simulink model "TwoDSimSimpleAero1stGen"  (R2021b)
settings: Solver=VariableStepAuto  StartTime=0.0  StopTime=5  RelTol=1e-3
undefined symbols (not defined in the file): Dterm, Iterm, Pterm
libraries: simulink_extras x4, simulink x1, slpidlib x1
settings Model: Creator=Andres  LastModifiedBy=Andres
settings SolverCC: ZeroCrossAlgorithm=Adaptive
settings DebuggingCC: AlgebraicLoopMsg=none  IgnoredZcDiagnostic=none

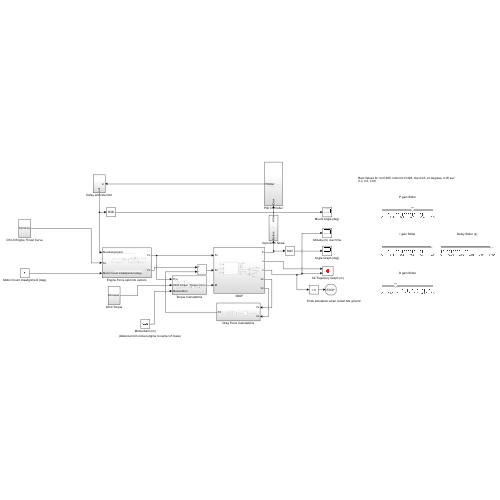
[thumbnail: Simulink's stored preview of the top-level diagram]
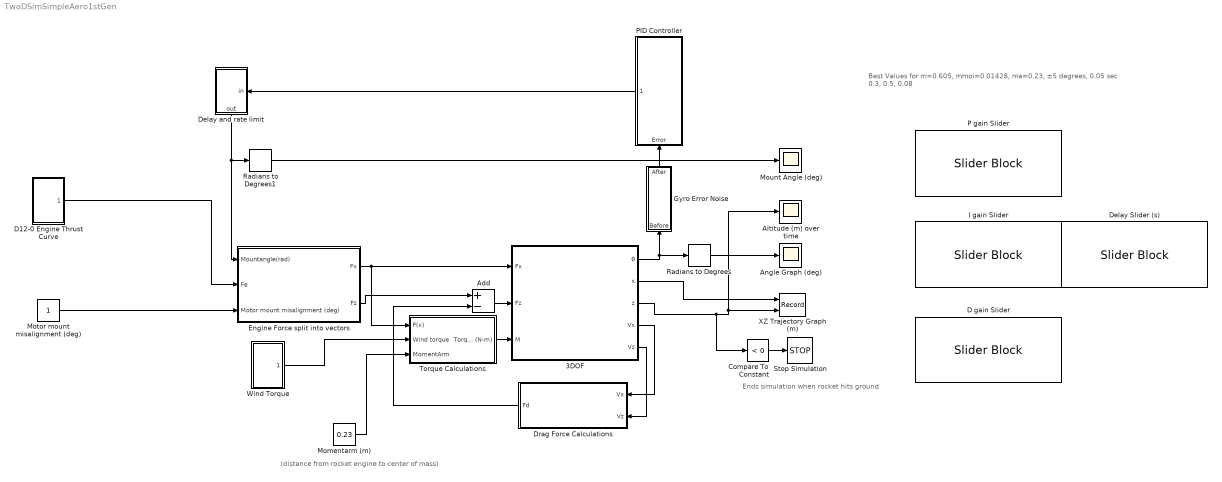
== system TwoDSimSimpleAero1stGen ==
  note: Best Values for m=0.605, mmoi=0.01428, ma=0.23, ±5 degrees, 0.05 sec
      | 0.3, 0.5, 0.08
  note: Ends simulation when rocket hits ground
  note: (distance from rocket engine to center of mass)
  3DOF : Subsystem
  Add : Sum  Inputs=+-
  Altitude (m) over time : Scope
  Angle Graph (deg) : Scope
  Compare To Constant : simulink/Logic and Bit Operations/Compare To Constant  relop=<  const=0  OutDataTypeStr=boolean
  D gain Slider : SliderBlock  LabelPosition=Hide  ScaleMax=0.3
  D12-0 Engine Thrust Curve : Subsystem
  Delay Slider (s) : SliderBlock  LabelPosition=Hide  ScaleMax=0.05  TickInterval=0.01
  Delay and rate limit : Subsystem
      settings: PortSchema="{\"entries\":[{\"content\":{\"sides\":[{\"content\":{\"connectorIds\":[\"In1\"]},\"type\":\"ConnectorPlacement.EquallySpacedRectSide\",\"uuid\":\"7f945310-91d5-4a5b-a152-cb378cea97e0\"},{\"content\":{\"connectorIds\":[],\"side\":\"RIGHT\"},\"type\":\"ConnectorPlacement.EquallySpacedRectSide\",\"uuid\":\"570eb395-808b-402d-8169-834796957515\"},{\"content\":{\"connectorIds\":[],\"side\":\"TOP\"},\"type\":\"ConnectorPlacement.EquallySpacedRectSide\",\"uuid\":\"f414d9f5-06db-41f9-9870-e73b040f5e14\"},{\"content\":{\"connectorIds\":[\"Out1\"],\"side\":\"BOTTOM\"},\"type\":\"ConnectorPlacement.EquallySpacedRectSide\",\"uuid\":\"dd3ad95d-53d5-4309-a4ef-7403eee50954\"}]},\"type\":\"ConnectorPlacement.EquallySpacedConnector\",\"uuid\":\"16f64462-feef-497e-ac9f-2db815891e61\"}],\"packageUris\":[\"http://schema.mathworks.com/mf0/Connector/R2020b\"],\"version\":\"1.0\"}"
  Drag Force Calculations : Subsystem
  Engine Force split into vectors : Subsystem
  Gyro Error Noise : Subsystem
      settings: PortSchema="{\"entries\":[{\"content\":{\"sides\":[{\"content\":{\"connectorIds\":[]},\"type\":\"ConnectorPlacement.EquallySpacedRectSide\",\"uuid\":\"db613b74-a95a-4e78-b0b5-852c38ce090d\"},{\"content\":{\"connectorIds\":[],\"side\":\"RIGHT\"},\"type\":\"ConnectorPlacement.EquallySpacedRectSide\",\"uuid\":\"8ff7bb38-cc09-4562-ae4b-2277c61965ca\"},{\"content\":{\"connectorIds\":[\"Out1\"],\"side\":\"TOP\"},\"type\":\"ConnectorPlacement.EquallySpacedRectSide\",\"uuid\":\"fa7b536e-f18b-43ee-b35a-7562f98f0dcc\"},{\"content\":{\"connectorIds\":[\"In1\"],\"side\":\"BOTTOM\"},\"type\":\"ConnectorPlacement.EquallySpacedRectSide\",\"uuid\":\"dd72ef68-23e3-4e8c-8031-36f0d8372741\"}]},\"type\":\"ConnectorPlacement.EquallySpacedConnector\",\"uuid\":\"56970b38-3c02-4837-94fb-dc8b3090c774\"}],\"packageUris\":[\"http://schema.mathworks.com/mf0/Connector/R2020b\"],\"version\":\"1.0\"}"
  I gain Slider : SliderBlock  LabelPosition=Hide  ScaleMax=0.5
  Momentarm (m) : Constant  Value=0.23
  Motor mount misalignment (deg) : Constant
  Mount Angle (deg) : Scope
  P gain Slider : SliderBlock  LabelPosition=Hide  ScaleMax=0.5
  PID Controller : Subsystem
      settings: PortSchema="{\"entries\":[{\"content\":{\"sides\":[{\"content\":{\"connectorIds\":[\"Out1\"]},\"type\":\"ConnectorPlacement.EquallySpacedRectSide\",\"uuid\":\"3056940d-b626-4ad3-aea6-cbabeac63329\"},{\"content\":{\"connectorIds\":[],\"side\":\"RIGHT\"},\"type\":\"ConnectorPlacement.EquallySpacedRectSide\",\"uuid\":\"0510cd9b-8fa4-4f8a-80ec-38231d972233\"},{\"content\":{\"connectorIds\":[],\"side\":\"TOP\"},\"type\":\"ConnectorPlacement.EquallySpacedRectSide\",\"uuid\":\"9c9a70ab-b090-41d6-ac7a-a7598bc3d7a5\"},{\"content\":{\"connectorIds\":[\"In1\"],\"side\":\"BOTTOM\"},\"type\":\"ConnectorPlacement.EquallySpacedRectSide\",\"uuid\":\"76047b82-5909-4180-a207-d443029300af\"}]},\"type\":\"ConnectorPlacement.EquallySpacedConnector\",\"uuid\":\"ba61792f-c506-461f-9738-365393edbd5c\"}],\"packageUris\":[\"http://schema.mathworks.com/mf0/Connector/R2020b\"],\"version\":\"1.0\"}"
  Radians to Degrees : simulink_extras/Transformations/Radians to Degrees
  Radians to Degrees1 : simulink_extras/Transformations/Radians to Degrees
  Stop Simulation : Stop
  Torque Calculations : Subsystem
  Wind Torque : Subsystem
  XZ Trajectory Graph (m) : Record  FileSettingsInternal="{\"entries\":[{\"content\":{\"excelSettings\":{\"content\":{},\"type\":\"Streamout.ExcelSettings\"}},\"type\":\"Streamout.FileSettingStorage\",\"uuid\":\"b17d18d2-045f-4c2f-bb1f-32f760d49c3f\"}],\"packageUris\":[\"http://schema.mathworks.com/mf0/streamout_blocks/R2020a\"],\"version\":\"1.0\"}"  Layout=[1 1]  SignalsInternal="{\"entries\":[{\"content\":{\"signals\":[{\"content\":{\"blockPath\":[\"TwoDSimSimpleAero1stGen/XZ Trajectory Graph (m)\"],\"channel\":[],\"dimensions\":[1],\"domain\":\"TwoDSimSimpleAero1stGen/XZ Trajectory Graph (m)\",\"lineColor\":\"#fe330a\",\"plots\":[1],\"port\":1,\"sid\":[\"\"],\"signalID\":81,\"signalName\":\"3DOF:2\"},\"type\":\"RecordBlkView.Signal\",\"uuid\":\"15905c86-6a6c-439f-aa8f-17a391bc4a57\"},{\"content\":{\"blockPath\":[\"TwoDSimSimpleAero1stGen/XZ Trajectory Graph (m)\"],\"channel\":[],\"dimensions\":[1],\"domain\":\"TwoDSimSimpleAero1stGen/XZ Trajectory Graph (m)\",\"lineColor\":\"#22b573\",\"plots\":[1],\"port\":2,\"sid\":[\"\"],\"signalID\":85,\"signalName\":\"3DOF:3\"},\"type\":\"RecordBlkView.Signal\",\"uuid\":\"f1bda5b5-dd59-48e2-bdf2-818b15901255\"}]},\"type\":\"RecordBlkView.InputSignals\",\"uuid\":\"d9778f91-fdcf-43d5-b0d8-99f691514bf1\"}],\"packageUris\":[\"http://schema.mathworks.com/mf0/streamout_blocks/R2020a\"],\"version\":\"1.0\"}"  VisualizationBindings="{\"xyplotplugin\":{\"info\":[{\"series\":[{\"bindingParametersList\":[{\"parameter\":\"X-Axis\",\"signalID\":81,\"signalName\":\"3DOF:2\"},{\"parameter\":\"Y-Axis\",\"signalID\":85,\"signalName\":\"3DOF:3\"}],\"seriesID\":63584}],\"subplotID\":1}]}}"  CompatibilityTag=XY
  wires:
  3DOF/3(z) -> Altitude (m) over time/1, XZ Trajectory Graph (m)/2, Compare To Constant/1
  Compare To Constant/1 -> Stop Simulation/1
  3DOF/2(x) -> XZ Trajectory Graph (m)/1
  Motor mount misalignment (deg)/1 -> Engine Force split into vectors/3(Motor mount misalignment (deg))
  D12-0 Engine Thrust Curve/1(F(D12-0)) -> Engine Force split into vectors/2(Fe)
  Gyro Error Noise/1(After) -> PID Controller/1(Error)
  Delay and rate limit/1(out) -> Engine Force split into vectors/1(Mountangle(rad)), Radians to Degrees1/1
  Momentarm (m)/1 -> Torque Calculations/3(MomentArm)
  Radians to Degrees1/1 -> Mount Angle (deg)/1
  Engine Force split into vectors/2(Fz) -> Add/1
  Engine Force split into vectors/1(Fx) -> 3DOF/1(Fx), Torque Calculations/1(F(x))
  Drag Force Calculations/1(Fd) -> Add/2
  3DOF/1(" θ") -> Radians to Degrees/1, Gyro Error Noise/1(Before)
  Add/1 -> 3DOF/2(Fz)
  Torque Calculations/1(Torque (N-m)) -> 3DOF/3(M)
  3DOF/4(Vx) -> Drag Force Calculations/1(Vx)
  3DOF/5(Vz) -> Drag Force Calculations/2(Vz)
  Radians to Degrees/1 -> Angle Graph (deg)/1
  PID Controller/1(PIDOut) -> Delay and rate limit/1(in)
  Wind Torque/1(Wind torque) -> Torque Calculations/2(Wind torque)

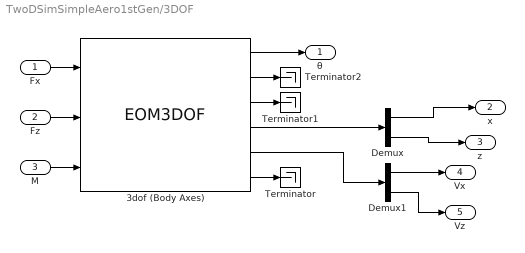
== system TwoDSimSimpleAero1stGen/3DOF ==
  Fx : Inport
  Fz : Inport  Port=2
  M : Inport  Port=3
  3dof (Body Axes) : EOM3DOF  v_ini=0.00000000000000000001  pos_ini=[0 0.1]  mass=0.605  Iyy=0.01428  g=-9.81
  Demux : Demux  Outputs=2
  Demux1 : Demux  Outputs=2
  Terminator : Terminator
  Terminator1 : Terminator
  Terminator2 : Terminator
  " θ" : Outport
  x : Outport  Port=2
  z : Outport  Port=3
  Vx : Outport  Port=4
  Vz : Outport  Port=5
  wires:
  Fz/1 -> 3dof (Body Axes)/2
  3dof (Body Axes)/2 -> Terminator2/1
  3dof (Body Axes)/6 -> Terminator/1
  Fx/1 -> 3dof (Body Axes)/1
  3dof (Body Axes)/3 -> Terminator1/1
  M/1 -> 3dof (Body Axes)/3
  3dof (Body Axes)/1 -> " θ"/1
  3dof (Body Axes)/4 -> Demux/1
  Demux/1 -> x/1
  Demux/2 -> z/1
  3dof (Body Axes)/5 -> Demux1/1
  Demux1/1 -> Vx/1
  Demux1/2 -> Vz/1

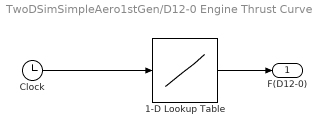
== system TwoDSimSimpleAero1stGen/D12-0 Engine Thrust Curve ==
  1-D Lookup Table : Lookup_n-D  NumberOfTableDimensions=1  BreakpointsForDimension1=[0 0.049 0.116 0.184 0.237 0.282 0.297 0.311 0.322 0.348 0.386 0.442 0.546 0.718 0.879 1.066 1.257 1.436 1.59 1.612 1.65]  Table=[0 2.569 9.369 17.275 24.258 29.73 27.01 22.589 17.99 14.126 12.099 10.808 9.876 9.306 9.105 8.901 8.698 8.31 8.294 4.613 0]  ExtrapMethod=Clip  UseLastTableValue=on  InternalRulePriority=Speed  RndMeth=Nearest  InputSameDT=on
  Clock : Clock
  F(D12-0) : Outport
  wires:
  Clock/1 -> 1-D Lookup Table/1
  1-D Lookup Table/1 -> F(D12-0)/1

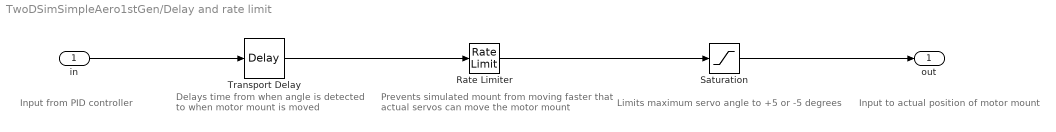
== system TwoDSimSimpleAero1stGen/Delay and rate limit ==
  note: Input to actual position of motor mount
  note: Input from PID controller
  note: Limits maximum servo angle to +5 or -5 degrees
  note: Prevents simulated mount from moving faster
      | that actual servos can move the motor mount
  note: Delays time from when angle is
      | detected to when motor mount is moved
  in : Inport
  Rate Limiter : RateLimiter  RisingSlewLimit=4.5  FallingSlewLimit=-4.5  SampleTimeMode=inherited
  Saturation : Saturate  UpperLimit=0.0872665  LowerLimit=-0.0872665
  Transport Delay : TransportDelay  DelayTime=0.05
  out : Outport
  wires:
  Transport Delay/1 -> Rate Limiter/1
  in/1 -> Transport Delay/1
  Rate Limiter/1 -> Saturation/1
  Saturation/1 -> out/1

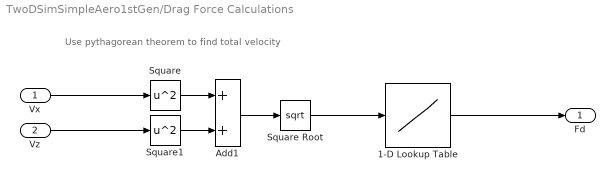
== system TwoDSimSimpleAero1stGen/Drag Force Calculations ==
  note: Use pythagorean theorem to find total velocity
  Vx : Inport
  Vz : Inport  Port=2
  1-D Lookup Table : Lookup_n-D  NumberOfTableDimensions=1  BreakpointsForDimension1=|  Table=|  InternalRulePriority=Speed  RndMeth=Simplest  InputSameDT=on
      BreakpointsForDimension1=|
      | [0
      | 0.10097
      | 0.59821
      | 1.53
      | 2.9145
      | 4.0886
      | 4.5849
      | 4.9184
      | 5.1856
      | 5.4204
      | 5.6288
      | 5.8251
      | 6.01
      | 6.1838
      | 6.3516
      | 6.5153
      | 6.675
      | 6.8309
      | 6.9833
      | 7.1323
      | 7.2776
      | 7.4196
      | 7.5581
      | 7.6931
      | 7.8242
      | 7.9484
      | 8.0652
      | 8.1745
      | 8.2794
      | 8.3842
      | 8.489]
      Table=|
      | [0
      | 1.81E-05
      | 5.00E-04
      | 0.0027243
      | 0.0089101
      | 0.016699
      | 0.020672
      | 0.023564
      | 0.02601
      | 0.028253
      | 0.030318
      | 0.032326
      | 0.034272
      | 0.036151
      | 0.038009
      | 0.039865
      | 0.041716
      | 0.043561
      | 0.045401
      | 0.047234
      | 0.049056
      | 0.050867
      | 0.052663
      | 0.054443
      | 0.056198
      | 0.057885
      | 0.059492
      | 0.061015
      | 0.062494
      | 0.063988
      | 0.065499]
  Add1 : Sum
  Square : Math  Operator=square  SaturateOnIntegerOverflow=on
  Square Root : Sqrt  SaturateOnIntegerOverflow=on
  Square1 : Math  Operator=square  SaturateOnIntegerOverflow=on
  Fd : Outport
  wires:
  Square1/1 -> Add1/2
  Vx/1 -> Square/1
  Square Root/1 -> 1-D Lookup Table/1
  Add1/1 -> Square Root/1
  Square/1 -> Add1/1
  Vz/1 -> Square1/1
  1-D Lookup Table/1 -> Fd/1

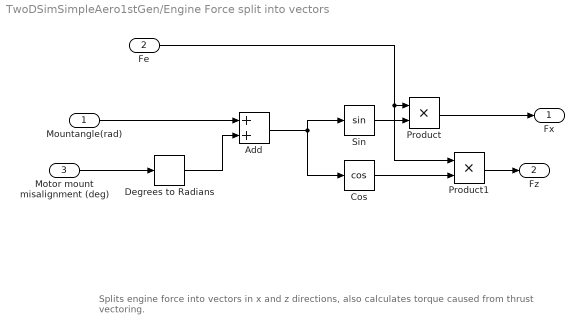
== system TwoDSimSimpleAero1stGen/Engine Force split into vectors ==
  note: Splits engine force into vectors in x and z directions, also calculates torque caused from thrust vectoring.
  Mountangle(rad) : Inport
  Fe : Inport  Port=2
  Motor mount misalignment (deg) : Inport  Port=3
  Add : Sum
  Cos : Trigonometry  Operator=cos
  Degrees to Radians : simulink_extras/Transformations/Degrees to Radians
  Product : Product
  Product1 : Product
  Sin : Trigonometry
  Fx : Outport
  Fz : Outport  Port=2
  wires:
  Sin/1 -> Product/2
  Product1/1 -> Fz/1
  Cos/1 -> Product1/2
  Product/1 -> Fx/1
  Fe/1 -> Product1/1, Product/1
  Mountangle(rad)/1 -> Add/1
  Add/1 -> Cos/1, Sin/1
  Degrees to Radians/1 -> Add/2
  Motor mount misalignment (deg)/1 -> Degrees to Radians/1

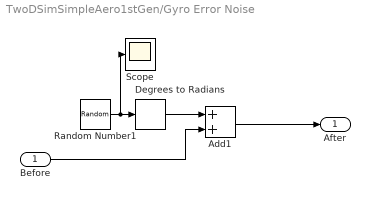
== system TwoDSimSimpleAero1stGen/Gyro Error Noise ==
  Before : Inport
  Add1 : Sum
  Degrees to Radians : simulink_extras/Transformations/Degrees to Radians
  Random Number1 : RandomNumber  Variance=0.01  SampleTime=0.1
  Scope : Scope
  After : Outport
  wires:
  Degrees to Radians/1 -> Add1/1
  Before/1 -> Add1/2
  Random Number1/1 -> Scope/1, Degrees to Radians/1
  Add1/1 -> After/1

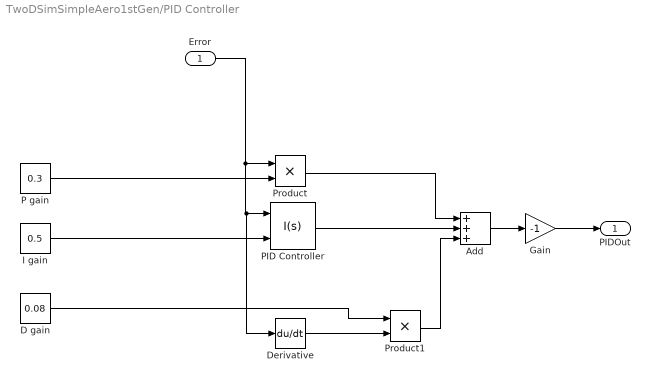
== system TwoDSimSimpleAero1stGen/PID Controller ==
  Error : Inport
  Add : Sum  Inputs=+++
  D gain : Constant  Value=0.08
  Derivative : Derivative
  Gain : Gain  Gain=-1
  I gain : Constant  Value=0.5
  P gain : Constant  Value=0.3
  PID Controller : slpidlib/PID Controller  Controller=I  Form=Parallel  TimeDomain=Continuous-time  UseExternalTs=off  SampleTime=-1  IntegratorMethod=Forward Euler  FilterMethod=Forward Euler  ControllerParametersSource=external  P=Pterm  I=Iterm  D=Dterm  UseFilter=on  N=100  TunerSelectOption=Transfer Function Based (PID Tuner App)  InitialConditionSource=internal  InitialConditionForIntegrator=0  InitialConditionForFilter=0  DifferentiatorICPrevScaledInput=0  ExternalReset=none  TrackingMode=off  Kt=1  LimitOutput=off  SatLimitsSource=internal  UpperSaturationLimit=inf  LowerSaturationLimit=-inf  LinearizeAsGain=on  AntiWindupMode=none  Kb=1  POutMin=[]  POutMax=[]  IOutMin=[]  IOutMax=[]  DOutMin=[]  DOutMax=[]  NOutMin=[]  NOutMax=[]  SumOutMin=[]  SumOutMax=[]  SaturationOutMin=[]  SaturationOutMax=[]  PParamMin=[]  PParamMax=[]  IParamMin=[]  IParamMax=[]  DParamMin=[]  DParamMax=[]  NParamMin=[]  NParamMax=[]  KbParamMin=[]  KbParamMax=[]  KtParamMin=[]  KtParamMax=[]  KbOutMin=[]  KbOutMax=[]  KtOutMin=[]  KtOutMax=[]  IntegratorOutMin=[]  IntegratorOutMax=[]  FilterOutMin=[]  FilterOutMax=[]  SumI1OutMin=[]  SumI1OutMax=[]  SumI2OutMin=[]  SumI2OutMax=[]  SumI3OutMin=[]  SumI3OutMax=[]  SumI4OutMin=[]  SumI4OutMax=[]  SumDOutMin=[]  SumDOutMax=[]  DifferentiatorOutMin=[]  DifferentiatorOutMax=[]  FilterDiffOutCoefMin=[]  FilterDiffOutCoefMax=[]  ReciprocalOutMin=[]  ReciprocalOutMax=[]  SumDenOutMin=[]  SumDenOutMax=[]  SumNumOutMin=[]  SumNumOutMax=[]  DivideOutMin=[]  DivideOutMax=[]  UdiffTsProdOutMin=[]  UdiffTsProdOutMax=[]  NTsProdOutMin=[]  NTsProdOutMax=[]  UintegralTsProdOutMin=[]  UintegralTsProdOutMax=[]  UngainTsProdOutMin=[]  UngainTsProdOutMax=[]  IntegratorContinuousStateAttributes=''  IntegratorStateMustResolveToSignalObject=off  IntegratorRTWStateStorageClass=Auto  FilterContinuousStateAttributes=''  FilterStateMustResolveToSignalObject=off  FilterRTWStateStorageClass=Auto  ParallelPVariant=Disabled  IdealPVariant=Disabled  IVariant=ExternalParameters  DVariant=Disabled  IntegratorVariant=Continuous  SatVariant=Disabled  AWVariant=Passthrough  PCopyVariant=Disabled  TRVariant=Disabled  FdbkBlocksVariant=Forward  IdealPFdbkVariant=Disabled  SatFdbkVariant=Disabled  DerivativeFilterVariant=Disabled  NVariant=Disabled  NCopyVariant=Disabled_SignalSpec  FilterICVariant=Disabled  IntegratorICVariant=InternalICs  ExternalResetVariant=Disabled  TRSumVariant=Passthrough  SumFdbkVariant=Disabled  SumVariant=Passthrough_I  TsampFilterVariant=InternalTs  TsampNgainVariant=Passthrough  TsampIntegralVariant=Passthrough  ExternalSaturationOutDataTypeStr=Inherit: Same as second input
  Product : Product
  Product1 : Product
  PIDOut : Outport
  wires:
  Error/1 -> Derivative/1, PID Controller/1, Product/1
  Gain/1 -> PIDOut/1
  Add/1 -> Gain/1
  Product/1 -> Add/1
  PID Controller/1 -> Add/2
  P gain/1 -> Product/2
  Derivative/1 -> Product1/2
  Product1/1 -> Add/3
  I gain/1 -> PID Controller/2
  D gain/1 -> Product1/1

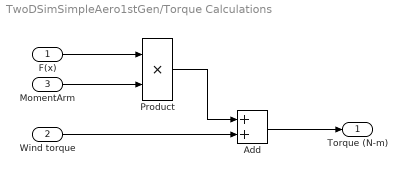
== system TwoDSimSimpleAero1stGen/Torque Calculations ==
  F(x) : Inport
  Wind torque : Inport  Port=2
  MomentArm : Inport  Port=3
  Add : Sum
  Product : Product
  Torque (N-m) : Outport
  wires:
  Add/1 -> Torque (N-m)/1
  F(x)/1 -> Product/1
  MomentArm/1 -> Product/2
  Product/1 -> Add/1
  Wind torque/1 -> Add/2

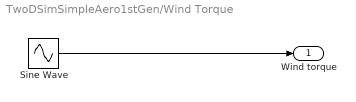
== system TwoDSimSimpleAero1stGen/Wind Torque ==
  Sine Wave : Sin  Amplitude=0.05  Bias=0.1  Frequency=2.5  SampleTime=0
  Wind torque : Outport
  wires:
  Sine Wave/1 -> Wind torque/1
